simulink model "car_pendulum_control"  (R2020b)
settings: Solver=VariableStepAuto  StartTime=0.0  StopTime=6  RelTol=1e-3
settings Model: Creator=petir  LastModifiedBy=petir

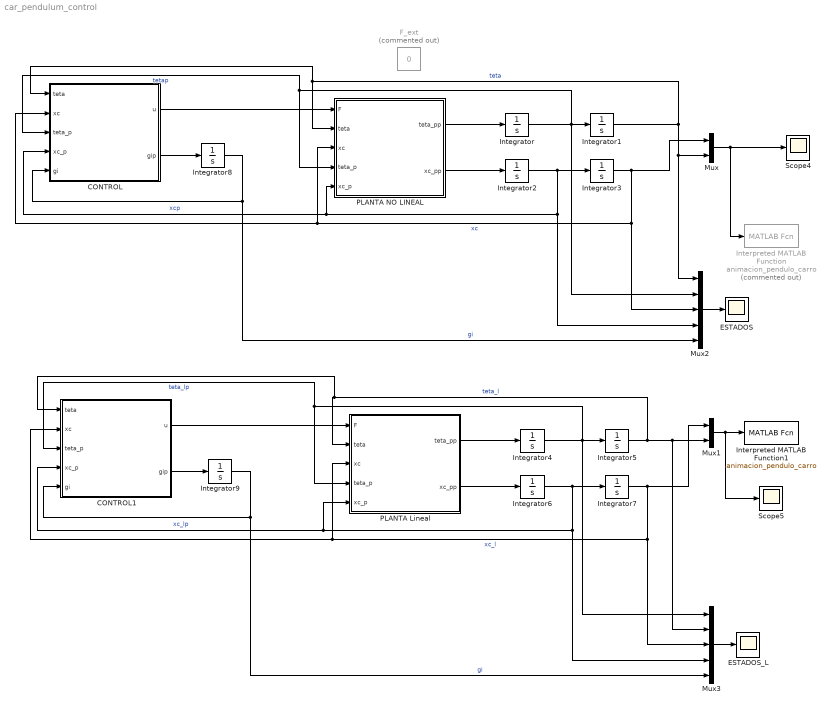
== system car_pendulum_control ==
  CONTROL : MATLAB Function  TreatAsAtomicUnit=on
  CONTROL1 : MATLAB Function  TreatAsAtomicUnit=on
  ESTADOS : Scope
  ESTADOS_L : Scope
  F_ext : Constant  Commented=on  Value=0
  Integrator{,1..9} (10 alike) : Integrator
  Interpreted MATLAB Function : MATLABFcn  Commented=on  MATLABFcn=animacion_pendulo_carro  OutputDimensions=0
  Interpreted MATLAB Function1 : MATLABFcn  MATLABFcn=animacion_pendulo_carro  OutputDimensions=0
  Mux : Mux  Inputs=2
  Mux1 : Mux  Inputs=2
  Mux2 : Mux  Inputs=5
  Mux3 : Mux  Inputs=5
  PLANTA Lineal : MATLAB Function  TreatAsAtomicUnit=on
  PLANTA NO LINEAL : MATLAB Function  TreatAsAtomicUnit=on
  Scope4 : Scope
  Scope5 : Scope
  wires:
  PLANTA NO LINEAL/1(teta_pp) -> Integrator/1
  Integrator/1 -> PLANTA NO LINEAL/4(teta_p), CONTROL/3(teta_p), Integrator1/1, Mux2/2  "tetap"
  Integrator1/1 -> Mux2/1, Mux/2, PLANTA NO LINEAL/2(teta), CONTROL/1(teta)  "teta"
  PLANTA NO LINEAL/2(xc_pp) -> Integrator2/1
  Integrator2/1 -> CONTROL/4(xc_p), PLANTA NO LINEAL/5(xc_p), Mux2/4, Integrator3/1  "xcp"
  Integrator3/1 -> Mux2/3, CONTROL/2(xc), PLANTA NO LINEAL/3(xc), Mux/1  "xc"
  PLANTA Lineal/2(xc_pp) -> Integrator6/1
  Integrator6/1 -> Mux3/4, PLANTA Lineal/5(xc_p), CONTROL1/4(xc_p), Integrator7/1  "xc_lp"
  Integrator4/1 -> CONTROL1/3(teta_p), PLANTA Lineal/4(teta_p), Mux3/1, Integrator5/1  "teta_lp"
  Integrator5/1 -> Mux3/2, Mux1/2, CONTROL1/1(teta), PLANTA Lineal/2(teta)  "teta_l"
  Integrator7/1 -> Mux3/3, CONTROL1/2(xc), PLANTA Lineal/3(xc), Mux1/1  "xc_l"
  PLANTA Lineal/1(teta_pp) -> Integrator4/1
  Mux/1 -> Scope4/1, Interpreted MATLAB Function/1
  Mux1/1 -> Scope5/1, Interpreted MATLAB Function1/1
  CONTROL/1(u) -> PLANTA NO LINEAL/1(F)
  CONTROL/2(gip) -> Integrator8/1
  Integrator8/1 -> Mux2/5, CONTROL/5(gi)  "gi"
  Mux2/1 -> ESTADOS/1
  CONTROL1/2(gip) -> Integrator9/1
  Integrator9/1 -> Mux3/5, CONTROL1/5(gi)  "gi"
  CONTROL1/1(u) -> PLANTA Lineal/1(F)
  Mux3/1 -> ESTADOS_L/1

== matlab function car_pendulum_control/PLANTA Lineal ==
  data: F input; teta_pp output; teta input; xc input; teta_p input; xc_p input; xc_pp output
function [teta_pp, xc_pp] = fcn(F, teta, xc, teta_p, xc_p)
m = 1;
M = 2;
l = 0.5;
L = 1;
g = 9.81;

% sin(teta) ~= 0
% xc_pp = F / (M + 2*m);
% teta_pp = -F / (l * (M + 2*m));

% sin(teta) ~= teta
% xc_pp = (F - m * g * teta) / M;
% teta_pp = (-F + (M + m) * g * teta) / M;

A = [0, 1, 0, 0; 
    (M+m)*g/(M*l), 0, 0, 0; 
    0, 0, 0, 1; 
    -m*g/M, 0, 0, 0];
B=[0; -1/(M*l); 0;  1/M];
X = [teta; teta_p; xc; xc_p];
Y = A*X + B*F;
teta_pp = Y(2);
xc_pp = Y(4);

== matlab function car_pendulum_control/PLANTA NO LINEAL ==
  data: F input; teta_pp output; teta input; xc input; teta_p input; xc_p input; xc_pp output
function [teta_pp, xc_pp] = fcn(F, teta, xc, teta_p, xc_p)
m = 1;
M = 2;
l = 0.5;
L = 1;
g = 9.81;

det = ((M + m)*m*l^2 - (m*l*cos(teta))^2);

xc_pp = (m*l^2 * (F + m*l*sin(teta) * teta_p^2)... 
            - m*l*cos(teta) * (m*g*l*sin(teta))) / det;
teta_pp = (-m*l*cos(teta) * (F + m*l*sin(teta) * teta_p^2)...
            + (M + m)*(m*g*l*sin(teta))) / det;

== matlab function car_pendulum_control/CONTROL ==
  data: teta input; xc input; teta_p input; xc_p input; gi input; u output; gip output
function [u, gip] = fcn(teta, xc, teta_p, xc_p, gi)
% Plant
M = 2;
m = 0.1; 
L = 0.5;
g = 9.81;
% Reference
r = 1;

A = [0 , 1, 0, 0; 
    (M+m)*g/(M*L), 0, 0, 0;
    0, 0, 0, 1;
    -m*g/M, 0, 0, 0];
B = [0; -1/(M*L); 0; 1/M];
C = [0, 0, 1, 0];

K = [-157.633619775739,-35.3733027419025,-56.0652395514781,-36.7466054838049];
Ki = -50.968399592252790;

% AA = [A-B*K, B*Ki; -C, 0];
% BB = [0; 0; 0; 0; 1];
% CC = [C 0];
% DD = [0]

X = [teta; teta_p; xc; xc_p];
Y = C * X;

u = -K * X + Ki*gi;
gip = r - Y;

== matlab function car_pendulum_control/CONTROL1 ==
  data: teta input; xc input; teta_p input; xc_p input; gi input; u output; gip output
function [u, gip] = fcn(teta, xc, teta_p, xc_p, gi)
% Plant
M = 2;
m = 0.1; 
L = 0.5;
g = 9.81;
% Reference
r = 1;

A = [0 , 1, 0, 0; 
    (M+m)*g/(M*L), 0, 0, 0;
    0, 0, 0, 1;
    -m*g/M, 0, 0, 0];
B = [0; -1/(M*L); 0; 1/M];
C = [0, 0, 1, 0];

K = [-157.633619775739,-35.3733027419025,-56.0652395514781,-36.7466054838049];
Ki = -50.968399592252790;

% AA = [A-B*K, B*Ki; -C, 0];
% BB = [0; 0; 0; 0; 1];
% CC = [C 0];
% DD = [0]

X = [teta; teta_p; xc; xc_p];
Y = C * X;

u = -K * X + Ki*gi;
gip = r - Y;
